simulink model "gm_parallel_lht_vnl"  (R2019b)
settings: Solver=FixedStepDiscrete  StartTime=0.0  StopTime=inf  RelTol=1e-3
undefined symbols (not defined in the file or in its folder): bt, height, nTheta, width
libraries: hdlsllib x199, simulink x27, hdlmdlgenlib x7, dspsrcs4 x1
(part 18 of 19)

== system gm_parallel_lht_vnl/Parallel LHT/Parallel LHT Kernel/Hough Kernel/Hough Kernel Symmetric Look Ahead/Look Ahead Hough/Register Bank_instance32 ==
  Data In : Inport  OutDataTypeStr=fixdt(1, 9, 0)  PortDimensions=1  SampleTime=6.66666666666667e-09
  Write Enable : Inport  Port=2  OutDataTypeStr=boolean  PortDimensions=1  SampleTime=6.66666666666667e-09
  Delay_Switch : Switch  Criteria=u2 ~= 0  Threshold=double(0)  OutDataTypeStr=fixdt(1, 9, 0)  SampleTime=6.66666666666667e-09
  Unit Delay Enabled Synchronous_lowered : Delay  DelayLength=double(1)  InitialCondition=0  SampleTime=6.66666666666667e-09
  Data Out : Outport
  wires:
  Unit Delay Enabled Synchronous_lowered/1 -> Data Out/1, Delay_Switch/3
  Data In/1 -> Delay_Switch/1
  Write Enable/1 -> Delay_Switch/2
  Delay_Switch/1 -> Unit Delay Enabled Synchronous_lowered/1

== system gm_parallel_lht_vnl/Parallel LHT/Parallel LHT Kernel/Hough Kernel/Hough Kernel Symmetric Look Ahead/Look Ahead Hough/Register Bank_instance33 ==
  Data In : Inport  OutDataTypeStr=fixdt(1, 9, 0)  PortDimensions=1  SampleTime=6.66666666666667e-09
  Write Enable : Inport  Port=2  OutDataTypeStr=boolean  PortDimensions=1  SampleTime=6.66666666666667e-09
  Delay_Switch : Switch  Criteria=u2 ~= 0  Threshold=double(0)  OutDataTypeStr=fixdt(1, 9, 0)  SampleTime=6.66666666666667e-09
  Unit Delay Enabled Synchronous_lowered : Delay  DelayLength=double(1)  InitialCondition=0  SampleTime=6.66666666666667e-09
  Data Out : Outport
  wires:
  Unit Delay Enabled Synchronous_lowered/1 -> Data Out/1, Delay_Switch/3
  Data In/1 -> Delay_Switch/1
  Write Enable/1 -> Delay_Switch/2
  Delay_Switch/1 -> Unit Delay Enabled Synchronous_lowered/1

== system gm_parallel_lht_vnl/Parallel LHT/Parallel LHT Kernel/Hough Kernel/Hough Kernel Symmetric Look Ahead/Look Ahead Hough/Register Bank_instance34 ==
  Data In : Inport  OutDataTypeStr=fixdt(1, 9, 0)  PortDimensions=1  SampleTime=6.66666666666667e-09
  Write Enable : Inport  Port=2  OutDataTypeStr=boolean  PortDimensions=1  SampleTime=6.66666666666667e-09
  Delay_Switch : Switch  Criteria=u2 ~= 0  Threshold=double(0)  OutDataTypeStr=fixdt(1, 9, 0)  SampleTime=6.66666666666667e-09
  Unit Delay Enabled Synchronous_lowered : Delay  DelayLength=double(1)  InitialCondition=0  SampleTime=6.66666666666667e-09
  Data Out : Outport
  wires:
  Unit Delay Enabled Synchronous_lowered/1 -> Data Out/1, Delay_Switch/3
  Data In/1 -> Delay_Switch/1
  Write Enable/1 -> Delay_Switch/2
  Delay_Switch/1 -> Unit Delay Enabled Synchronous_lowered/1

== system gm_parallel_lht_vnl/Parallel LHT/Parallel LHT Kernel/Hough Kernel/Hough Kernel Symmetric Look Ahead/Look Ahead Hough/Register Bank_instance35 ==
  Data In : Inport  OutDataTypeStr=fixdt(1, 9, 0)  PortDimensions=1  SampleTime=6.66666666666667e-09
  Write Enable : Inport  Port=2  OutDataTypeStr=boolean  PortDimensions=1  SampleTime=6.66666666666667e-09
  Delay_Switch : Switch  Criteria=u2 ~= 0  Threshold=double(0)  OutDataTypeStr=fixdt(1, 9, 0)  SampleTime=6.66666666666667e-09
  Unit Delay Enabled Synchronous_lowered : Delay  DelayLength=double(1)  InitialCondition=0  SampleTime=6.66666666666667e-09
  Data Out : Outport
  wires:
  Unit Delay Enabled Synchronous_lowered/1 -> Data Out/1, Delay_Switch/3
  Data In/1 -> Delay_Switch/1
  Write Enable/1 -> Delay_Switch/2
  Delay_Switch/1 -> Unit Delay Enabled Synchronous_lowered/1

== system gm_parallel_lht_vnl/Parallel LHT/Parallel LHT Kernel/Hough Kernel/Hough Kernel Symmetric Look Ahead/Look Ahead Hough/Register Bank_instance36 ==
  Data In : Inport  OutDataTypeStr=fixdt(1, 9, 0)  PortDimensions=1  SampleTime=6.66666666666667e-09
  Write Enable : Inport  Port=2  OutDataTypeStr=boolean  PortDimensions=1  SampleTime=6.66666666666667e-09
  Delay_Switch : Switch  Criteria=u2 ~= 0  Threshold=double(0)  OutDataTypeStr=fixdt(1, 9, 0)  SampleTime=6.66666666666667e-09
  Unit Delay Enabled Synchronous_lowered : Delay  DelayLength=double(1)  InitialCondition=0  SampleTime=6.66666666666667e-09
  Data Out : Outport
  wires:
  Unit Delay Enabled Synchronous_lowered/1 -> Data Out/1, Delay_Switch/3
  Data In/1 -> Delay_Switch/1
  Write Enable/1 -> Delay_Switch/2
  Delay_Switch/1 -> Unit Delay Enabled Synchronous_lowered/1

== system gm_parallel_lht_vnl/Parallel LHT/Parallel LHT Kernel/Hough Kernel/Hough Kernel Symmetric Look Ahead/Look Ahead Hough/Register Bank_instance37 ==
  Data In : Inport  OutDataTypeStr=fixdt(1, 9, 0)  PortDimensions=1  SampleTime=6.66666666666667e-09
  Write Enable : Inport  Port=2  OutDataTypeStr=boolean  PortDimensions=1  SampleTime=6.66666666666667e-09
  Delay_Switch : Switch  Criteria=u2 ~= 0  Threshold=double(0)  OutDataTypeStr=fixdt(1, 9, 0)  SampleTime=6.66666666666667e-09
  Unit Delay Enabled Synchronous_lowered : Delay  DelayLength=double(1)  InitialCondition=0  SampleTime=6.66666666666667e-09
  Data Out : Outport
  wires:
  Unit Delay Enabled Synchronous_lowered/1 -> Data Out/1, Delay_Switch/3
  Data In/1 -> Delay_Switch/1
  Write Enable/1 -> Delay_Switch/2
  Delay_Switch/1 -> Unit Delay Enabled Synchronous_lowered/1

== system gm_parallel_lht_vnl/Parallel LHT/Parallel LHT Kernel/Hough Kernel/Hough Kernel Symmetric Look Ahead/Look Ahead Hough/Register Bank_instance38 ==
  Data In : Inport  OutDataTypeStr=fixdt(1, 9, 0)  PortDimensions=1  SampleTime=6.66666666666667e-09
  Write Enable : Inport  Port=2  OutDataTypeStr=boolean  PortDimensions=1  SampleTime=6.66666666666667e-09
  Delay_Switch : Switch  Criteria=u2 ~= 0  Threshold=double(0)  OutDataTypeStr=fixdt(1, 9, 0)  SampleTime=6.66666666666667e-09
  Unit Delay Enabled Synchronous_lowered : Delay  DelayLength=double(1)  InitialCondition=0  SampleTime=6.66666666666667e-09
  Data Out : Outport
  wires:
  Unit Delay Enabled Synchronous_lowered/1 -> Data Out/1, Delay_Switch/3
  Data In/1 -> Delay_Switch/1
  Write Enable/1 -> Delay_Switch/2
  Delay_Switch/1 -> Unit Delay Enabled Synchronous_lowered/1

== system gm_parallel_lht_vnl/Parallel LHT/Parallel LHT Kernel/Hough Kernel/Hough Kernel Symmetric Look Ahead/Look Ahead Hough/Register Bank_instance39 ==
  Data In : Inport  OutDataTypeStr=fixdt(1, 9, 0)  PortDimensions=1  SampleTime=6.66666666666667e-09
  Write Enable : Inport  Port=2  OutDataTypeStr=boolean  PortDimensions=1  SampleTime=6.66666666666667e-09
  Delay_Switch : Switch  Criteria=u2 ~= 0  Threshold=double(0)  OutDataTypeStr=fixdt(1, 9, 0)  SampleTime=6.66666666666667e-09
  Unit Delay Enabled Synchronous_lowered : Delay  DelayLength=double(1)  InitialCondition=0  SampleTime=6.66666666666667e-09
  Data Out : Outport
  wires:
  Unit Delay Enabled Synchronous_lowered/1 -> Data Out/1, Delay_Switch/3
  Data In/1 -> Delay_Switch/1
  Write Enable/1 -> Delay_Switch/2
  Delay_Switch/1 -> Unit Delay Enabled Synchronous_lowered/1

== system gm_parallel_lht_vnl/Parallel LHT/Parallel LHT Kernel/Hough Kernel/Hough Kernel Symmetric Look Ahead/Look Ahead Hough/Register Bank_instance4 ==
  Data In : Inport  OutDataTypeStr=fixdt(1, 9, 0)  PortDimensions=1  SampleTime=6.66666666666667e-09
  Write Enable : Inport  Port=2  OutDataTypeStr=boolean  PortDimensions=1  SampleTime=6.66666666666667e-09
  Delay_Switch : Switch  Criteria=u2 ~= 0  Threshold=double(0)  OutDataTypeStr=fixdt(1, 9, 0)  SampleTime=6.66666666666667e-09
  Unit Delay Enabled Synchronous_lowered : Delay  DelayLength=double(1)  InitialCondition=0  SampleTime=6.66666666666667e-09
  Data Out : Outport
  wires:
  Unit Delay Enabled Synchronous_lowered/1 -> Data Out/1, Delay_Switch/3
  Data In/1 -> Delay_Switch/1
  Write Enable/1 -> Delay_Switch/2
  Delay_Switch/1 -> Unit Delay Enabled Synchronous_lowered/1

== system gm_parallel_lht_vnl/Parallel LHT/Parallel LHT Kernel/Hough Kernel/Hough Kernel Symmetric Look Ahead/Look Ahead Hough/Register Bank_instance40 ==
  Data In : Inport  OutDataTypeStr=fixdt(1, 9, 0)  PortDimensions=1  SampleTime=6.66666666666667e-09
  Write Enable : Inport  Port=2  OutDataTypeStr=boolean  PortDimensions=1  SampleTime=6.66666666666667e-09
  Delay_Switch : Switch  Criteria=u2 ~= 0  Threshold=double(0)  OutDataTypeStr=fixdt(1, 9, 0)  SampleTime=6.66666666666667e-09
  Unit Delay Enabled Synchronous_lowered : Delay  DelayLength=double(1)  InitialCondition=0  SampleTime=6.66666666666667e-09
  Data Out : Outport
  wires:
  Unit Delay Enabled Synchronous_lowered/1 -> Data Out/1, Delay_Switch/3
  Data In/1 -> Delay_Switch/1
  Write Enable/1 -> Delay_Switch/2
  Delay_Switch/1 -> Unit Delay Enabled Synchronous_lowered/1

== system gm_parallel_lht_vnl/Parallel LHT/Parallel LHT Kernel/Hough Kernel/Hough Kernel Symmetric Look Ahead/Look Ahead Hough/Register Bank_instance41 ==
  Data In : Inport  OutDataTypeStr=fixdt(1, 9, 0)  PortDimensions=1  SampleTime=6.66666666666667e-09
  Write Enable : Inport  Port=2  OutDataTypeStr=boolean  PortDimensions=1  SampleTime=6.66666666666667e-09
  Delay_Switch : Switch  Criteria=u2 ~= 0  Threshold=double(0)  OutDataTypeStr=fixdt(1, 9, 0)  SampleTime=6.66666666666667e-09
  Unit Delay Enabled Synchronous_lowered : Delay  DelayLength=double(1)  InitialCondition=0  SampleTime=6.66666666666667e-09
  Data Out : Outport
  wires:
  Unit Delay Enabled Synchronous_lowered/1 -> Data Out/1, Delay_Switch/3
  Data In/1 -> Delay_Switch/1
  Write Enable/1 -> Delay_Switch/2
  Delay_Switch/1 -> Unit Delay Enabled Synchronous_lowered/1

== system gm_parallel_lht_vnl/Parallel LHT/Parallel LHT Kernel/Hough Kernel/Hough Kernel Symmetric Look Ahead/Look Ahead Hough/Register Bank_instance42 ==
  Data In : Inport  OutDataTypeStr=fixdt(1, 9, 0)  PortDimensions=1  SampleTime=6.66666666666667e-09
  Write Enable : Inport  Port=2  OutDataTypeStr=boolean  PortDimensions=1  SampleTime=6.66666666666667e-09
  Delay_Switch : Switch  Criteria=u2 ~= 0  Threshold=double(0)  OutDataTypeStr=fixdt(1, 9, 0)  SampleTime=6.66666666666667e-09
  Unit Delay Enabled Synchronous_lowered : Delay  DelayLength=double(1)  InitialCondition=0  SampleTime=6.66666666666667e-09
  Data Out : Outport
  wires:
  Unit Delay Enabled Synchronous_lowered/1 -> Data Out/1, Delay_Switch/3
  Data In/1 -> Delay_Switch/1
  Write Enable/1 -> Delay_Switch/2
  Delay_Switch/1 -> Unit Delay Enabled Synchronous_lowered/1

== system gm_parallel_lht_vnl/Parallel LHT/Parallel LHT Kernel/Hough Kernel/Hough Kernel Symmetric Look Ahead/Look Ahead Hough/Register Bank_instance43 ==
  Data In : Inport  OutDataTypeStr=fixdt(1, 9, 0)  PortDimensions=1  SampleTime=6.66666666666667e-09
  Write Enable : Inport  Port=2  OutDataTypeStr=boolean  PortDimensions=1  SampleTime=6.66666666666667e-09
  Delay_Switch : Switch  Criteria=u2 ~= 0  Threshold=double(0)  OutDataTypeStr=fixdt(1, 9, 0)  SampleTime=6.66666666666667e-09
  Unit Delay Enabled Synchronous_lowered : Delay  DelayLength=double(1)  InitialCondition=0  SampleTime=6.66666666666667e-09
  Data Out : Outport
  wires:
  Unit Delay Enabled Synchronous_lowered/1 -> Data Out/1, Delay_Switch/3
  Data In/1 -> Delay_Switch/1
  Write Enable/1 -> Delay_Switch/2
  Delay_Switch/1 -> Unit Delay Enabled Synchronous_lowered/1

== system gm_parallel_lht_vnl/Parallel LHT/Parallel LHT Kernel/Hough Kernel/Hough Kernel Symmetric Look Ahead/Look Ahead Hough/Register Bank_instance44 ==
  Data In : Inport  OutDataTypeStr=fixdt(1, 9, 0)  PortDimensions=1  SampleTime=6.66666666666667e-09
  Write Enable : Inport  Port=2  OutDataTypeStr=boolean  PortDimensions=1  SampleTime=6.66666666666667e-09
  Delay_Switch : Switch  Criteria=u2 ~= 0  Threshold=double(0)  OutDataTypeStr=fixdt(1, 9, 0)  SampleTime=6.66666666666667e-09
  Unit Delay Enabled Synchronous_lowered : Delay  DelayLength=double(1)  InitialCondition=0  SampleTime=6.66666666666667e-09
  Data Out : Outport
  wires:
  Unit Delay Enabled Synchronous_lowered/1 -> Data Out/1, Delay_Switch/3
  Data In/1 -> Delay_Switch/1
  Write Enable/1 -> Delay_Switch/2
  Delay_Switch/1 -> Unit Delay Enabled Synchronous_lowered/1

== system gm_parallel_lht_vnl/Parallel LHT/Parallel LHT Kernel/Hough Kernel/Hough Kernel Symmetric Look Ahead/Look Ahead Hough/Register Bank_instance45 ==
  Data In : Inport  OutDataTypeStr=fixdt(1, 9, 0)  PortDimensions=1  SampleTime=6.66666666666667e-09
  Write Enable : Inport  Port=2  OutDataTypeStr=boolean  PortDimensions=1  SampleTime=6.66666666666667e-09
  Delay_Switch : Switch  Criteria=u2 ~= 0  Threshold=double(0)  OutDataTypeStr=fixdt(1, 9, 0)  SampleTime=6.66666666666667e-09
  Unit Delay Enabled Synchronous_lowered : Delay  DelayLength=double(1)  InitialCondition=0  SampleTime=6.66666666666667e-09
  Data Out : Outport
  wires:
  Unit Delay Enabled Synchronous_lowered/1 -> Data Out/1, Delay_Switch/3
  Data In/1 -> Delay_Switch/1
  Write Enable/1 -> Delay_Switch/2
  Delay_Switch/1 -> Unit Delay Enabled Synchronous_lowered/1

== system gm_parallel_lht_vnl/Parallel LHT/Parallel LHT Kernel/Hough Kernel/Hough Kernel Symmetric Look Ahead/Look Ahead Hough/Register Bank_instance46 ==
  Data In : Inport  OutDataTypeStr=fixdt(1, 9, 0)  PortDimensions=1  SampleTime=6.66666666666667e-09
  Write Enable : Inport  Port=2  OutDataTypeStr=boolean  PortDimensions=1  SampleTime=6.66666666666667e-09
  Delay_Switch : Switch  Criteria=u2 ~= 0  Threshold=double(0)  OutDataTypeStr=fixdt(1, 9, 0)  SampleTime=6.66666666666667e-09
  Unit Delay Enabled Synchronous_lowered : Delay  DelayLength=double(1)  InitialCondition=0  SampleTime=6.66666666666667e-09
  Data Out : Outport
  wires:
  Unit Delay Enabled Synchronous_lowered/1 -> Data Out/1, Delay_Switch/3
  Data In/1 -> Delay_Switch/1
  Write Enable/1 -> Delay_Switch/2
  Delay_Switch/1 -> Unit Delay Enabled Synchronous_lowered/1

== system gm_parallel_lht_vnl/Parallel LHT/Parallel LHT Kernel/Hough Kernel/Hough Kernel Symmetric Look Ahead/Look Ahead Hough/Register Bank_instance47 ==
  Data In : Inport  OutDataTypeStr=fixdt(1, 9, 0)  PortDimensions=1  SampleTime=6.66666666666667e-09
  Write Enable : Inport  Port=2  OutDataTypeStr=boolean  PortDimensions=1  SampleTime=6.66666666666667e-09
  Delay_Switch : Switch  Criteria=u2 ~= 0  Threshold=double(0)  OutDataTypeStr=fixdt(1, 9, 0)  SampleTime=6.66666666666667e-09
  Unit Delay Enabled Synchronous_lowered : Delay  DelayLength=double(1)  InitialCondition=0  SampleTime=6.66666666666667e-09
  Data Out : Outport
  wires:
  Unit Delay Enabled Synchronous_lowered/1 -> Data Out/1, Delay_Switch/3
  Data In/1 -> Delay_Switch/1
  Write Enable/1 -> Delay_Switch/2
  Delay_Switch/1 -> Unit Delay Enabled Synchronous_lowered/1

== system gm_parallel_lht_vnl/Parallel LHT/Parallel LHT Kernel/Hough Kernel/Hough Kernel Symmetric Look Ahead/Look Ahead Hough/Register Bank_instance48 ==
  Data In : Inport  OutDataTypeStr=fixdt(1, 9, 0)  PortDimensions=1  SampleTime=6.66666666666667e-09
  Write Enable : Inport  Port=2  OutDataTypeStr=boolean  PortDimensions=1  SampleTime=6.66666666666667e-09
  Delay_Switch : Switch  Criteria=u2 ~= 0  Threshold=double(0)  OutDataTypeStr=fixdt(1, 9, 0)  SampleTime=6.66666666666667e-09
  Unit Delay Enabled Synchronous_lowered : Delay  DelayLength=double(1)  InitialCondition=0  SampleTime=6.66666666666667e-09
  Data Out : Outport
  wires:
  Unit Delay Enabled Synchronous_lowered/1 -> Data Out/1, Delay_Switch/3
  Data In/1 -> Delay_Switch/1
  Write Enable/1 -> Delay_Switch/2
  Delay_Switch/1 -> Unit Delay Enabled Synchronous_lowered/1

== system gm_parallel_lht_vnl/Parallel LHT/Parallel LHT Kernel/Hough Kernel/Hough Kernel Symmetric Look Ahead/Look Ahead Hough/Register Bank_instance49 ==
  Data In : Inport  OutDataTypeStr=fixdt(1, 9, 0)  PortDimensions=1  SampleTime=6.66666666666667e-09
  Write Enable : Inport  Port=2  OutDataTypeStr=boolean  PortDimensions=1  SampleTime=6.66666666666667e-09
  Delay_Switch : Switch  Criteria=u2 ~= 0  Threshold=double(0)  OutDataTypeStr=fixdt(1, 9, 0)  SampleTime=6.66666666666667e-09
  Unit Delay Enabled Synchronous_lowered : Delay  DelayLength=double(1)  InitialCondition=0  SampleTime=6.66666666666667e-09
  Data Out : Outport
  wires:
  Unit Delay Enabled Synchronous_lowered/1 -> Data Out/1, Delay_Switch/3
  Data In/1 -> Delay_Switch/1
  Write Enable/1 -> Delay_Switch/2
  Delay_Switch/1 -> Unit Delay Enabled Synchronous_lowered/1

== system gm_parallel_lht_vnl/Parallel LHT/Parallel LHT Kernel/Hough Kernel/Hough Kernel Symmetric Look Ahead/Look Ahead Hough/Register Bank_instance5 ==
  Data In : Inport  OutDataTypeStr=fixdt(1, 9, 0)  PortDimensions=1  SampleTime=6.66666666666667e-09
  Write Enable : Inport  Port=2  OutDataTypeStr=boolean  PortDimensions=1  SampleTime=6.66666666666667e-09
  Delay_Switch : Switch  Criteria=u2 ~= 0  Threshold=double(0)  OutDataTypeStr=fixdt(1, 9, 0)  SampleTime=6.66666666666667e-09
  Unit Delay Enabled Synchronous_lowered : Delay  DelayLength=double(1)  InitialCondition=0  SampleTime=6.66666666666667e-09
  Data Out : Outport
  wires:
  Unit Delay Enabled Synchronous_lowered/1 -> Data Out/1, Delay_Switch/3
  Data In/1 -> Delay_Switch/1
  Write Enable/1 -> Delay_Switch/2
  Delay_Switch/1 -> Unit Delay Enabled Synchronous_lowered/1

== system gm_parallel_lht_vnl/Parallel LHT/Parallel LHT Kernel/Hough Kernel/Hough Kernel Symmetric Look Ahead/Look Ahead Hough/Register Bank_instance50 ==
  Data In : Inport  OutDataTypeStr=fixdt(1, 9, 0)  PortDimensions=1  SampleTime=6.66666666666667e-09
  Write Enable : Inport  Port=2  OutDataTypeStr=boolean  PortDimensions=1  SampleTime=6.66666666666667e-09
  Delay_Switch : Switch  Criteria=u2 ~= 0  Threshold=double(0)  OutDataTypeStr=fixdt(1, 9, 0)  SampleTime=6.66666666666667e-09
  Unit Delay Enabled Synchronous_lowered : Delay  DelayLength=double(1)  InitialCondition=0  SampleTime=6.66666666666667e-09
  Data Out : Outport
  wires:
  Unit Delay Enabled Synchronous_lowered/1 -> Data Out/1, Delay_Switch/3
  Data In/1 -> Delay_Switch/1
  Write Enable/1 -> Delay_Switch/2
  Delay_Switch/1 -> Unit Delay Enabled Synchronous_lowered/1

== system gm_parallel_lht_vnl/Parallel LHT/Parallel LHT Kernel/Hough Kernel/Hough Kernel Symmetric Look Ahead/Look Ahead Hough/Register Bank_instance51 ==
  Data In : Inport  OutDataTypeStr=fixdt(1, 9, 0)  PortDimensions=1  SampleTime=6.66666666666667e-09
  Write Enable : Inport  Port=2  OutDataTypeStr=boolean  PortDimensions=1  SampleTime=6.66666666666667e-09
  Delay_Switch : Switch  Criteria=u2 ~= 0  Threshold=double(0)  OutDataTypeStr=fixdt(1, 9, 0)  SampleTime=6.66666666666667e-09
  Unit Delay Enabled Synchronous_lowered : Delay  DelayLength=double(1)  InitialCondition=0  SampleTime=6.66666666666667e-09
  Data Out : Outport
  wires:
  Unit Delay Enabled Synchronous_lowered/1 -> Data Out/1, Delay_Switch/3
  Data In/1 -> Delay_Switch/1
  Write Enable/1 -> Delay_Switch/2
  Delay_Switch/1 -> Unit Delay Enabled Synchronous_lowered/1

== system gm_parallel_lht_vnl/Parallel LHT/Parallel LHT Kernel/Hough Kernel/Hough Kernel Symmetric Look Ahead/Look Ahead Hough/Register Bank_instance52 ==
  Data In : Inport  OutDataTypeStr=fixdt(1, 9, 0)  PortDimensions=1  SampleTime=6.66666666666667e-09
  Write Enable : Inport  Port=2  OutDataTypeStr=boolean  PortDimensions=1  SampleTime=6.66666666666667e-09
  Delay_Switch : Switch  Criteria=u2 ~= 0  Threshold=double(0)  OutDataTypeStr=fixdt(1, 9, 0)  SampleTime=6.66666666666667e-09
  Unit Delay Enabled Synchronous_lowered : Delay  DelayLength=double(1)  InitialCondition=0  SampleTime=6.66666666666667e-09
  Data Out : Outport
  wires:
  Unit Delay Enabled Synchronous_lowered/1 -> Data Out/1, Delay_Switch/3
  Data In/1 -> Delay_Switch/1
  Write Enable/1 -> Delay_Switch/2
  Delay_Switch/1 -> Unit Delay Enabled Synchronous_lowered/1

== system gm_parallel_lht_vnl/Parallel LHT/Parallel LHT Kernel/Hough Kernel/Hough Kernel Symmetric Look Ahead/Look Ahead Hough/Register Bank_instance53 ==
  Data In : Inport  OutDataTypeStr=fixdt(1, 9, 0)  PortDimensions=1  SampleTime=6.66666666666667e-09
  Write Enable : Inport  Port=2  OutDataTypeStr=boolean  PortDimensions=1  SampleTime=6.66666666666667e-09
  Delay_Switch : Switch  Criteria=u2 ~= 0  Threshold=double(0)  OutDataTypeStr=fixdt(1, 9, 0)  SampleTime=6.66666666666667e-09
  Unit Delay Enabled Synchronous_lowered : Delay  DelayLength=double(1)  InitialCondition=0  SampleTime=6.66666666666667e-09
  Data Out : Outport
  wires:
  Unit Delay Enabled Synchronous_lowered/1 -> Data Out/1, Delay_Switch/3
  Data In/1 -> Delay_Switch/1
  Write Enable/1 -> Delay_Switch/2
  Delay_Switch/1 -> Unit Delay Enabled Synchronous_lowered/1

== system gm_parallel_lht_vnl/Parallel LHT/Parallel LHT Kernel/Hough Kernel/Hough Kernel Symmetric Look Ahead/Look Ahead Hough/Register Bank_instance54 ==
  Data In : Inport  OutDataTypeStr=fixdt(1, 9, 0)  PortDimensions=1  SampleTime=6.66666666666667e-09
  Write Enable : Inport  Port=2  OutDataTypeStr=boolean  PortDimensions=1  SampleTime=6.66666666666667e-09
  Delay_Switch : Switch  Criteria=u2 ~= 0  Threshold=double(0)  OutDataTypeStr=fixdt(1, 9, 0)  SampleTime=6.66666666666667e-09
  Unit Delay Enabled Synchronous_lowered : Delay  DelayLength=double(1)  InitialCondition=0  SampleTime=6.66666666666667e-09
  Data Out : Outport
  wires:
  Unit Delay Enabled Synchronous_lowered/1 -> Data Out/1, Delay_Switch/3
  Data In/1 -> Delay_Switch/1
  Write Enable/1 -> Delay_Switch/2
  Delay_Switch/1 -> Unit Delay Enabled Synchronous_lowered/1

== system gm_parallel_lht_vnl/Parallel LHT/Parallel LHT Kernel/Hough Kernel/Hough Kernel Symmetric Look Ahead/Look Ahead Hough/Register Bank_instance55 ==
  Data In : Inport  OutDataTypeStr=fixdt(1, 9, 0)  PortDimensions=1  SampleTime=6.66666666666667e-09
  Write Enable : Inport  Port=2  OutDataTypeStr=boolean  PortDimensions=1  SampleTime=6.66666666666667e-09
  Delay_Switch : Switch  Criteria=u2 ~= 0  Threshold=double(0)  OutDataTypeStr=fixdt(1, 9, 0)  SampleTime=6.66666666666667e-09
  Unit Delay Enabled Synchronous_lowered : Delay  DelayLength=double(1)  InitialCondition=0  SampleTime=6.66666666666667e-09
  Data Out : Outport
  wires:
  Unit Delay Enabled Synchronous_lowered/1 -> Data Out/1, Delay_Switch/3
  Data In/1 -> Delay_Switch/1
  Write Enable/1 -> Delay_Switch/2
  Delay_Switch/1 -> Unit Delay Enabled Synchronous_lowered/1

== system gm_parallel_lht_vnl/Parallel LHT/Parallel LHT Kernel/Hough Kernel/Hough Kernel Symmetric Look Ahead/Look Ahead Hough/Register Bank_instance56 ==
  Data In : Inport  OutDataTypeStr=fixdt(1, 9, 0)  PortDimensions=1  SampleTime=6.66666666666667e-09
  Write Enable : Inport  Port=2  OutDataTypeStr=boolean  PortDimensions=1  SampleTime=6.66666666666667e-09
  Delay_Switch : Switch  Criteria=u2 ~= 0  Threshold=double(0)  OutDataTypeStr=fixdt(1, 9, 0)  SampleTime=6.66666666666667e-09
  Unit Delay Enabled Synchronous_lowered : Delay  DelayLength=double(1)  InitialCondition=0  SampleTime=6.66666666666667e-09
  Data Out : Outport
  wires:
  Unit Delay Enabled Synchronous_lowered/1 -> Data Out/1, Delay_Switch/3
  Data In/1 -> Delay_Switch/1
  Write Enable/1 -> Delay_Switch/2
  Delay_Switch/1 -> Unit Delay Enabled Synchronous_lowered/1

== system gm_parallel_lht_vnl/Parallel LHT/Parallel LHT Kernel/Hough Kernel/Hough Kernel Symmetric Look Ahead/Look Ahead Hough/Register Bank_instance57 ==
  Data In : Inport  OutDataTypeStr=fixdt(1, 9, 0)  PortDimensions=1  SampleTime=6.66666666666667e-09
  Write Enable : Inport  Port=2  OutDataTypeStr=boolean  PortDimensions=1  SampleTime=6.66666666666667e-09
  Delay_Switch : Switch  Criteria=u2 ~= 0  Threshold=double(0)  OutDataTypeStr=fixdt(1, 9, 0)  SampleTime=6.66666666666667e-09
  Unit Delay Enabled Synchronous_lowered : Delay  DelayLength=double(1)  InitialCondition=0  SampleTime=6.66666666666667e-09
  Data Out : Outport
  wires:
  Unit Delay Enabled Synchronous_lowered/1 -> Data Out/1, Delay_Switch/3
  Data In/1 -> Delay_Switch/1
  Write Enable/1 -> Delay_Switch/2
  Delay_Switch/1 -> Unit Delay Enabled Synchronous_lowered/1

== system gm_parallel_lht_vnl/Parallel LHT/Parallel LHT Kernel/Hough Kernel/Hough Kernel Symmetric Look Ahead/Look Ahead Hough/Register Bank_instance58 ==
  Data In : Inport  OutDataTypeStr=fixdt(1, 9, 0)  PortDimensions=1  SampleTime=6.66666666666667e-09
  Write Enable : Inport  Port=2  OutDataTypeStr=boolean  PortDimensions=1  SampleTime=6.66666666666667e-09
  Delay_Switch : Switch  Criteria=u2 ~= 0  Threshold=double(0)  OutDataTypeStr=fixdt(1, 9, 0)  SampleTime=6.66666666666667e-09
  Unit Delay Enabled Synchronous_lowered : Delay  DelayLength=double(1)  InitialCondition=0  SampleTime=6.66666666666667e-09
  Data Out : Outport
  wires:
  Unit Delay Enabled Synchronous_lowered/1 -> Data Out/1, Delay_Switch/3
  Data In/1 -> Delay_Switch/1
  Write Enable/1 -> Delay_Switch/2
  Delay_Switch/1 -> Unit Delay Enabled Synchronous_lowered/1

== system gm_parallel_lht_vnl/Parallel LHT/Parallel LHT Kernel/Hough Kernel/Hough Kernel Symmetric Look Ahead/Look Ahead Hough/Register Bank_instance59 ==
  Data In : Inport  OutDataTypeStr=fixdt(1, 9, 0)  PortDimensions=1  SampleTime=6.66666666666667e-09
  Write Enable : Inport  Port=2  OutDataTypeStr=boolean  PortDimensions=1  SampleTime=6.66666666666667e-09
  Delay_Switch : Switch  Criteria=u2 ~= 0  Threshold=double(0)  OutDataTypeStr=fixdt(1, 9, 0)  SampleTime=6.66666666666667e-09
  Unit Delay Enabled Synchronous_lowered : Delay  DelayLength=double(1)  InitialCondition=0  SampleTime=6.66666666666667e-09
  Data Out : Outport
  wires:
  Unit Delay Enabled Synchronous_lowered/1 -> Data Out/1, Delay_Switch/3
  Data In/1 -> Delay_Switch/1
  Write Enable/1 -> Delay_Switch/2
  Delay_Switch/1 -> Unit Delay Enabled Synchronous_lowered/1

== system gm_parallel_lht_vnl/Parallel LHT/Parallel LHT Kernel/Hough Kernel/Hough Kernel Symmetric Look Ahead/Look Ahead Hough/Register Bank_instance6 ==
  Data In : Inport  OutDataTypeStr=fixdt(1, 9, 0)  PortDimensions=1  SampleTime=6.66666666666667e-09
  Write Enable : Inport  Port=2  OutDataTypeStr=boolean  PortDimensions=1  SampleTime=6.66666666666667e-09
  Delay_Switch : Switch  Criteria=u2 ~= 0  Threshold=double(0)  OutDataTypeStr=fixdt(1, 9, 0)  SampleTime=6.66666666666667e-09
  Unit Delay Enabled Synchronous_lowered : Delay  DelayLength=double(1)  InitialCondition=0  SampleTime=6.66666666666667e-09
  Data Out : Outport
  wires:
  Unit Delay Enabled Synchronous_lowered/1 -> Data Out/1, Delay_Switch/3
  Data In/1 -> Delay_Switch/1
  Write Enable/1 -> Delay_Switch/2
  Delay_Switch/1 -> Unit Delay Enabled Synchronous_lowered/1

== system gm_parallel_lht_vnl/Parallel LHT/Parallel LHT Kernel/Hough Kernel/Hough Kernel Symmetric Look Ahead/Look Ahead Hough/Register Bank_instance60 ==
  Data In : Inport  OutDataTypeStr=fixdt(1, 9, 0)  PortDimensions=1  SampleTime=6.66666666666667e-09
  Write Enable : Inport  Port=2  OutDataTypeStr=boolean  PortDimensions=1  SampleTime=6.66666666666667e-09
  Delay_Switch : Switch  Criteria=u2 ~= 0  Threshold=double(0)  OutDataTypeStr=fixdt(1, 9, 0)  SampleTime=6.66666666666667e-09
  Unit Delay Enabled Synchronous_lowered : Delay  DelayLength=double(1)  InitialCondition=0  SampleTime=6.66666666666667e-09
  Data Out : Outport
  wires:
  Unit Delay Enabled Synchronous_lowered/1 -> Data Out/1, Delay_Switch/3
  Data In/1 -> Delay_Switch/1
  Write Enable/1 -> Delay_Switch/2
  Delay_Switch/1 -> Unit Delay Enabled Synchronous_lowered/1

== system gm_parallel_lht_vnl/Parallel LHT/Parallel LHT Kernel/Hough Kernel/Hough Kernel Symmetric Look Ahead/Look Ahead Hough/Register Bank_instance61 ==
  Data In : Inport  OutDataTypeStr=fixdt(1, 9, 0)  PortDimensions=1  SampleTime=6.66666666666667e-09
  Write Enable : Inport  Port=2  OutDataTypeStr=boolean  PortDimensions=1  SampleTime=6.66666666666667e-09
  Delay_Switch : Switch  Criteria=u2 ~= 0  Threshold=double(0)  OutDataTypeStr=fixdt(1, 9, 0)  SampleTime=6.66666666666667e-09
  Unit Delay Enabled Synchronous_lowered : Delay  DelayLength=double(1)  InitialCondition=0  SampleTime=6.66666666666667e-09
  Data Out : Outport
  wires:
  Unit Delay Enabled Synchronous_lowered/1 -> Data Out/1, Delay_Switch/3
  Data In/1 -> Delay_Switch/1
  Write Enable/1 -> Delay_Switch/2
  Delay_Switch/1 -> Unit Delay Enabled Synchronous_lowered/1

== system gm_parallel_lht_vnl/Parallel LHT/Parallel LHT Kernel/Hough Kernel/Hough Kernel Symmetric Look Ahead/Look Ahead Hough/Register Bank_instance62 ==
  Data In : Inport  OutDataTypeStr=fixdt(1, 9, 0)  PortDimensions=1  SampleTime=6.66666666666667e-09
  Write Enable : Inport  Port=2  OutDataTypeStr=boolean  PortDimensions=1  SampleTime=6.66666666666667e-09
  Delay_Switch : Switch  Criteria=u2 ~= 0  Threshold=double(0)  OutDataTypeStr=fixdt(1, 9, 0)  SampleTime=6.66666666666667e-09
  Unit Delay Enabled Synchronous_lowered : Delay  DelayLength=double(1)  InitialCondition=0  SampleTime=6.66666666666667e-09
  Data Out : Outport
  wires:
  Unit Delay Enabled Synchronous_lowered/1 -> Data Out/1, Delay_Switch/3
  Data In/1 -> Delay_Switch/1
  Write Enable/1 -> Delay_Switch/2
  Delay_Switch/1 -> Unit Delay Enabled Synchronous_lowered/1

== system gm_parallel_lht_vnl/Parallel LHT/Parallel LHT Kernel/Hough Kernel/Hough Kernel Symmetric Look Ahead/Look Ahead Hough/Register Bank_instance63 ==
  Data In : Inport  OutDataTypeStr=fixdt(1, 9, 0)  PortDimensions=1  SampleTime=6.66666666666667e-09
  Write Enable : Inport  Port=2  OutDataTypeStr=boolean  PortDimensions=1  SampleTime=6.66666666666667e-09
  Delay_Switch : Switch  Criteria=u2 ~= 0  Threshold=double(0)  OutDataTypeStr=fixdt(1, 9, 0)  SampleTime=6.66666666666667e-09
  Unit Delay Enabled Synchronous_lowered : Delay  DelayLength=double(1)  InitialCondition=0  SampleTime=6.66666666666667e-09
  Data Out : Outport
  wires:
  Unit Delay Enabled Synchronous_lowered/1 -> Data Out/1, Delay_Switch/3
  Data In/1 -> Delay_Switch/1
  Write Enable/1 -> Delay_Switch/2
  Delay_Switch/1 -> Unit Delay Enabled Synchronous_lowered/1

== system gm_parallel_lht_vnl/Parallel LHT/Parallel LHT Kernel/Hough Kernel/Hough Kernel Symmetric Look Ahead/Look Ahead Hough/Register Bank_instance64 ==
  Data In : Inport  OutDataTypeStr=fixdt(1, 9, 0)  PortDimensions=1  SampleTime=6.66666666666667e-09
  Write Enable : Inport  Port=2  OutDataTypeStr=boolean  PortDimensions=1  SampleTime=6.66666666666667e-09
  Delay_Switch : Switch  Criteria=u2 ~= 0  Threshold=double(0)  OutDataTypeStr=fixdt(1, 9, 0)  SampleTime=6.66666666666667e-09
  Unit Delay Enabled Synchronous_lowered : Delay  DelayLength=double(1)  InitialCondition=0  SampleTime=6.66666666666667e-09
  Data Out : Outport
  wires:
  Unit Delay Enabled Synchronous_lowered/1 -> Data Out/1, Delay_Switch/3
  Data In/1 -> Delay_Switch/1
  Write Enable/1 -> Delay_Switch/2
  Delay_Switch/1 -> Unit Delay Enabled Synchronous_lowered/1

== system gm_parallel_lht_vnl/Parallel LHT/Parallel LHT Kernel/Hough Kernel/Hough Kernel Symmetric Look Ahead/Look Ahead Hough/Register Bank_instance65 ==
  Data In : Inport  OutDataTypeStr=fixdt(1, 9, 0)  PortDimensions=1  SampleTime=6.66666666666667e-09
  Write Enable : Inport  Port=2  OutDataTypeStr=boolean  PortDimensions=1  SampleTime=6.66666666666667e-09
  Delay_Switch : Switch  Criteria=u2 ~= 0  Threshold=double(0)  OutDataTypeStr=fixdt(1, 9, 0)  SampleTime=6.66666666666667e-09
  Unit Delay Enabled Synchronous_lowered : Delay  DelayLength=double(1)  InitialCondition=0  SampleTime=6.66666666666667e-09
  Data Out : Outport
  wires:
  Unit Delay Enabled Synchronous_lowered/1 -> Data Out/1, Delay_Switch/3
  Data In/1 -> Delay_Switch/1
  Write Enable/1 -> Delay_Switch/2
  Delay_Switch/1 -> Unit Delay Enabled Synchronous_lowered/1

== system gm_parallel_lht_vnl/Parallel LHT/Parallel LHT Kernel/Hough Kernel/Hough Kernel Symmetric Look Ahead/Look Ahead Hough/Register Bank_instance66 ==
  Data In : Inport  OutDataTypeStr=fixdt(1, 9, 0)  PortDimensions=1  SampleTime=6.66666666666667e-09
  Write Enable : Inport  Port=2  OutDataTypeStr=boolean  PortDimensions=1  SampleTime=6.66666666666667e-09
  Delay_Switch : Switch  Criteria=u2 ~= 0  Threshold=double(0)  OutDataTypeStr=fixdt(1, 9, 0)  SampleTime=6.66666666666667e-09
  Unit Delay Enabled Synchronous_lowered : Delay  DelayLength=double(1)  InitialCondition=0  SampleTime=6.66666666666667e-09
  Data Out : Outport
  wires:
  Unit Delay Enabled Synchronous_lowered/1 -> Data Out/1, Delay_Switch/3
  Data In/1 -> Delay_Switch/1
  Write Enable/1 -> Delay_Switch/2
  Delay_Switch/1 -> Unit Delay Enabled Synchronous_lowered/1

== system gm_parallel_lht_vnl/Parallel LHT/Parallel LHT Kernel/Hough Kernel/Hough Kernel Symmetric Look Ahead/Look Ahead Hough/Register Bank_instance67 ==
  Data In : Inport  OutDataTypeStr=fixdt(1, 9, 0)  PortDimensions=1  SampleTime=6.66666666666667e-09
  Write Enable : Inport  Port=2  OutDataTypeStr=boolean  PortDimensions=1  SampleTime=6.66666666666667e-09
  Delay_Switch : Switch  Criteria=u2 ~= 0  Threshold=double(0)  OutDataTypeStr=fixdt(1, 9, 0)  SampleTime=6.66666666666667e-09
  Unit Delay Enabled Synchronous_lowered : Delay  DelayLength=double(1)  InitialCondition=0  SampleTime=6.66666666666667e-09
  Data Out : Outport
  wires:
  Unit Delay Enabled Synchronous_lowered/1 -> Data Out/1, Delay_Switch/3
  Data In/1 -> Delay_Switch/1
  Write Enable/1 -> Delay_Switch/2
  Delay_Switch/1 -> Unit Delay Enabled Synchronous_lowered/1

== system gm_parallel_lht_vnl/Parallel LHT/Parallel LHT Kernel/Hough Kernel/Hough Kernel Symmetric Look Ahead/Look Ahead Hough/Register Bank_instance68 ==
  Data In : Inport  OutDataTypeStr=fixdt(1, 9, 0)  PortDimensions=1  SampleTime=6.66666666666667e-09
  Write Enable : Inport  Port=2  OutDataTypeStr=boolean  PortDimensions=1  SampleTime=6.66666666666667e-09
  Delay_Switch : Switch  Criteria=u2 ~= 0  Threshold=double(0)  OutDataTypeStr=fixdt(1, 9, 0)  SampleTime=6.66666666666667e-09
  Unit Delay Enabled Synchronous_lowered : Delay  DelayLength=double(1)  InitialCondition=0  SampleTime=6.66666666666667e-09
  Data Out : Outport
  wires:
  Unit Delay Enabled Synchronous_lowered/1 -> Data Out/1, Delay_Switch/3
  Data In/1 -> Delay_Switch/1
  Write Enable/1 -> Delay_Switch/2
  Delay_Switch/1 -> Unit Delay Enabled Synchronous_lowered/1

== system gm_parallel_lht_vnl/Parallel LHT/Parallel LHT Kernel/Hough Kernel/Hough Kernel Symmetric Look Ahead/Look Ahead Hough/Register Bank_instance69 ==
  Data In : Inport  OutDataTypeStr=fixdt(1, 9, 0)  PortDimensions=1  SampleTime=6.66666666666667e-09
  Write Enable : Inport  Port=2  OutDataTypeStr=boolean  PortDimensions=1  SampleTime=6.66666666666667e-09
  Delay_Switch : Switch  Criteria=u2 ~= 0  Threshold=double(0)  OutDataTypeStr=fixdt(1, 9, 0)  SampleTime=6.66666666666667e-09
  Unit Delay Enabled Synchronous_lowered : Delay  DelayLength=double(1)  InitialCondition=0  SampleTime=6.66666666666667e-09
  Data Out : Outport
  wires:
  Unit Delay Enabled Synchronous_lowered/1 -> Data Out/1, Delay_Switch/3
  Data In/1 -> Delay_Switch/1
  Write Enable/1 -> Delay_Switch/2
  Delay_Switch/1 -> Unit Delay Enabled Synchronous_lowered/1

== system gm_parallel_lht_vnl/Parallel LHT/Parallel LHT Kernel/Hough Kernel/Hough Kernel Symmetric Look Ahead/Look Ahead Hough/Register Bank_instance7 ==
  Data In : Inport  OutDataTypeStr=fixdt(1, 9, 0)  PortDimensions=1  SampleTime=6.66666666666667e-09
  Write Enable : Inport  Port=2  OutDataTypeStr=boolean  PortDimensions=1  SampleTime=6.66666666666667e-09
  Delay_Switch : Switch  Criteria=u2 ~= 0  Threshold=double(0)  OutDataTypeStr=fixdt(1, 9, 0)  SampleTime=6.66666666666667e-09
  Unit Delay Enabled Synchronous_lowered : Delay  DelayLength=double(1)  InitialCondition=0  SampleTime=6.66666666666667e-09
  Data Out : Outport
  wires:
  Unit Delay Enabled Synchronous_lowered/1 -> Data Out/1, Delay_Switch/3
  Data In/1 -> Delay_Switch/1
  Write Enable/1 -> Delay_Switch/2
  Delay_Switch/1 -> Unit Delay Enabled Synchronous_lowered/1

== system gm_parallel_lht_vnl/Parallel LHT/Parallel LHT Kernel/Hough Kernel/Hough Kernel Symmetric Look Ahead/Look Ahead Hough/Register Bank_instance70 ==
  Data In : Inport  OutDataTypeStr=fixdt(1, 9, 0)  PortDimensions=1  SampleTime=6.66666666666667e-09
  Write Enable : Inport  Port=2  OutDataTypeStr=boolean  PortDimensions=1  SampleTime=6.66666666666667e-09
  Delay_Switch : Switch  Criteria=u2 ~= 0  Threshold=double(0)  OutDataTypeStr=fixdt(1, 9, 0)  SampleTime=6.66666666666667e-09
  Unit Delay Enabled Synchronous_lowered : Delay  DelayLength=double(1)  InitialCondition=0  SampleTime=6.66666666666667e-09
  Data Out : Outport
  wires:
  Unit Delay Enabled Synchronous_lowered/1 -> Data Out/1, Delay_Switch/3
  Data In/1 -> Delay_Switch/1
  Write Enable/1 -> Delay_Switch/2
  Delay_Switch/1 -> Unit Delay Enabled Synchronous_lowered/1

== system gm_parallel_lht_vnl/Parallel LHT/Parallel LHT Kernel/Hough Kernel/Hough Kernel Symmetric Look Ahead/Look Ahead Hough/Register Bank_instance71 ==
  Data In : Inport  OutDataTypeStr=fixdt(1, 9, 0)  PortDimensions=1  SampleTime=6.66666666666667e-09
  Write Enable : Inport  Port=2  OutDataTypeStr=boolean  PortDimensions=1  SampleTime=6.66666666666667e-09
  Delay_Switch : Switch  Criteria=u2 ~= 0  Threshold=double(0)  OutDataTypeStr=fixdt(1, 9, 0)  SampleTime=6.66666666666667e-09
  Unit Delay Enabled Synchronous_lowered : Delay  DelayLength=double(1)  InitialCondition=0  SampleTime=6.66666666666667e-09
  Data Out : Outport
  wires:
  Unit Delay Enabled Synchronous_lowered/1 -> Data Out/1, Delay_Switch/3
  Data In/1 -> Delay_Switch/1
  Write Enable/1 -> Delay_Switch/2
  Delay_Switch/1 -> Unit Delay Enabled Synchronous_lowered/1

== system gm_parallel_lht_vnl/Parallel LHT/Parallel LHT Kernel/Hough Kernel/Hough Kernel Symmetric Look Ahead/Look Ahead Hough/Register Bank_instance72 ==
  Data In : Inport  OutDataTypeStr=fixdt(1, 9, 0)  PortDimensions=1  SampleTime=6.66666666666667e-09
  Write Enable : Inport  Port=2  OutDataTypeStr=boolean  PortDimensions=1  SampleTime=6.66666666666667e-09
  Delay_Switch : Switch  Criteria=u2 ~= 0  Threshold=double(0)  OutDataTypeStr=fixdt(1, 9, 0)  SampleTime=6.66666666666667e-09
  Unit Delay Enabled Synchronous_lowered : Delay  DelayLength=double(1)  InitialCondition=0  SampleTime=6.66666666666667e-09
  Data Out : Outport
  wires:
  Unit Delay Enabled Synchronous_lowered/1 -> Data Out/1, Delay_Switch/3
  Data In/1 -> Delay_Switch/1
  Write Enable/1 -> Delay_Switch/2
  Delay_Switch/1 -> Unit Delay Enabled Synchronous_lowered/1

== system gm_parallel_lht_vnl/Parallel LHT/Parallel LHT Kernel/Hough Kernel/Hough Kernel Symmetric Look Ahead/Look Ahead Hough/Register Bank_instance73 ==
  Data In : Inport  OutDataTypeStr=fixdt(1, 9, 0)  PortDimensions=1  SampleTime=6.66666666666667e-09
  Write Enable : Inport  Port=2  OutDataTypeStr=boolean  PortDimensions=1  SampleTime=6.66666666666667e-09
  Delay_Switch : Switch  Criteria=u2 ~= 0  Threshold=double(0)  OutDataTypeStr=fixdt(1, 9, 0)  SampleTime=6.66666666666667e-09
  Unit Delay Enabled Synchronous_lowered : Delay  DelayLength=double(1)  InitialCondition=0  SampleTime=6.66666666666667e-09
  Data Out : Outport
  wires:
  Unit Delay Enabled Synchronous_lowered/1 -> Data Out/1, Delay_Switch/3
  Data In/1 -> Delay_Switch/1
  Write Enable/1 -> Delay_Switch/2
  Delay_Switch/1 -> Unit Delay Enabled Synchronous_lowered/1

== system gm_parallel_lht_vnl/Parallel LHT/Parallel LHT Kernel/Hough Kernel/Hough Kernel Symmetric Look Ahead/Look Ahead Hough/Register Bank_instance74 ==
  Data In : Inport  OutDataTypeStr=fixdt(1, 9, 0)  PortDimensions=1  SampleTime=6.66666666666667e-09
  Write Enable : Inport  Port=2  OutDataTypeStr=boolean  PortDimensions=1  SampleTime=6.66666666666667e-09
  Delay_Switch : Switch  Criteria=u2 ~= 0  Threshold=double(0)  OutDataTypeStr=fixdt(1, 9, 0)  SampleTime=6.66666666666667e-09
  Unit Delay Enabled Synchronous_lowered : Delay  DelayLength=double(1)  InitialCondition=0  SampleTime=6.66666666666667e-09
  Data Out : Outport
  wires:
  Unit Delay Enabled Synchronous_lowered/1 -> Data Out/1, Delay_Switch/3
  Data In/1 -> Delay_Switch/1
  Write Enable/1 -> Delay_Switch/2
  Delay_Switch/1 -> Unit Delay Enabled Synchronous_lowered/1

== system gm_parallel_lht_vnl/Parallel LHT/Parallel LHT Kernel/Hough Kernel/Hough Kernel Symmetric Look Ahead/Look Ahead Hough/Register Bank_instance75 ==
  Data In : Inport  OutDataTypeStr=fixdt(1, 9, 0)  PortDimensions=1  SampleTime=6.66666666666667e-09
  Write Enable : Inport  Port=2  OutDataTypeStr=boolean  PortDimensions=1  SampleTime=6.66666666666667e-09
  Delay_Switch : Switch  Criteria=u2 ~= 0  Threshold=double(0)  OutDataTypeStr=fixdt(1, 9, 0)  SampleTime=6.66666666666667e-09
  Unit Delay Enabled Synchronous_lowered : Delay  DelayLength=double(1)  InitialCondition=0  SampleTime=6.66666666666667e-09
  Data Out : Outport
  wires:
  Unit Delay Enabled Synchronous_lowered/1 -> Data Out/1, Delay_Switch/3
  Data In/1 -> Delay_Switch/1
  Write Enable/1 -> Delay_Switch/2
  Delay_Switch/1 -> Unit Delay Enabled Synchronous_lowered/1

== system gm_parallel_lht_vnl/Parallel LHT/Parallel LHT Kernel/Hough Kernel/Hough Kernel Symmetric Look Ahead/Look Ahead Hough/Register Bank_instance76 ==
  Data In : Inport  OutDataTypeStr=fixdt(1, 9, 0)  PortDimensions=1  SampleTime=6.66666666666667e-09
  Write Enable : Inport  Port=2  OutDataTypeStr=boolean  PortDimensions=1  SampleTime=6.66666666666667e-09
  Delay_Switch : Switch  Criteria=u2 ~= 0  Threshold=double(0)  OutDataTypeStr=fixdt(1, 9, 0)  SampleTime=6.66666666666667e-09
  Unit Delay Enabled Synchronous_lowered : Delay  DelayLength=double(1)  InitialCondition=0  SampleTime=6.66666666666667e-09
  Data Out : Outport
  wires:
  Unit Delay Enabled Synchronous_lowered/1 -> Data Out/1, Delay_Switch/3
  Data In/1 -> Delay_Switch/1
  Write Enable/1 -> Delay_Switch/2
  Delay_Switch/1 -> Unit Delay Enabled Synchronous_lowered/1

== system gm_parallel_lht_vnl/Parallel LHT/Parallel LHT Kernel/Hough Kernel/Hough Kernel Symmetric Look Ahead/Look Ahead Hough/Register Bank_instance77 ==
  Data In : Inport  OutDataTypeStr=fixdt(1, 9, 0)  PortDimensions=1  SampleTime=6.66666666666667e-09
  Write Enable : Inport  Port=2  OutDataTypeStr=boolean  PortDimensions=1  SampleTime=6.66666666666667e-09
  Delay_Switch : Switch  Criteria=u2 ~= 0  Threshold=double(0)  OutDataTypeStr=fixdt(1, 9, 0)  SampleTime=6.66666666666667e-09
  Unit Delay Enabled Synchronous_lowered : Delay  DelayLength=double(1)  InitialCondition=0  SampleTime=6.66666666666667e-09
  Data Out : Outport
  wires:
  Unit Delay Enabled Synchronous_lowered/1 -> Data Out/1, Delay_Switch/3
  Data In/1 -> Delay_Switch/1
  Write Enable/1 -> Delay_Switch/2
  Delay_Switch/1 -> Unit Delay Enabled Synchronous_lowered/1

== system gm_parallel_lht_vnl/Parallel LHT/Parallel LHT Kernel/Hough Kernel/Hough Kernel Symmetric Look Ahead/Look Ahead Hough/Register Bank_instance78 ==
  Data In : Inport  OutDataTypeStr=fixdt(1, 9, 0)  PortDimensions=1  SampleTime=6.66666666666667e-09
  Write Enable : Inport  Port=2  OutDataTypeStr=boolean  PortDimensions=1  SampleTime=6.66666666666667e-09
  Delay_Switch : Switch  Criteria=u2 ~= 0  Threshold=double(0)  OutDataTypeStr=fixdt(1, 9, 0)  SampleTime=6.66666666666667e-09
  Unit Delay Enabled Synchronous_lowered : Delay  DelayLength=double(1)  InitialCondition=0  SampleTime=6.66666666666667e-09
  Data Out : Outport
  wires:
  Unit Delay Enabled Synchronous_lowered/1 -> Data Out/1, Delay_Switch/3
  Data In/1 -> Delay_Switch/1
  Write Enable/1 -> Delay_Switch/2
  Delay_Switch/1 -> Unit Delay Enabled Synchronous_lowered/1

== system gm_parallel_lht_vnl/Parallel LHT/Parallel LHT Kernel/Hough Kernel/Hough Kernel Symmetric Look Ahead/Look Ahead Hough/Register Bank_instance79 ==
  Data In : Inport  OutDataTypeStr=fixdt(1, 9, 0)  PortDimensions=1  SampleTime=6.66666666666667e-09
  Write Enable : Inport  Port=2  OutDataTypeStr=boolean  PortDimensions=1  SampleTime=6.66666666666667e-09
  Delay_Switch : Switch  Criteria=u2 ~= 0  Threshold=double(0)  OutDataTypeStr=fixdt(1, 9, 0)  SampleTime=6.66666666666667e-09
  Unit Delay Enabled Synchronous_lowered : Delay  DelayLength=double(1)  InitialCondition=0  SampleTime=6.66666666666667e-09
  Data Out : Outport
  wires:
  Unit Delay Enabled Synchronous_lowered/1 -> Data Out/1, Delay_Switch/3
  Data In/1 -> Delay_Switch/1
  Write Enable/1 -> Delay_Switch/2
  Delay_Switch/1 -> Unit Delay Enabled Synchronous_lowered/1

== system gm_parallel_lht_vnl/Parallel LHT/Parallel LHT Kernel/Hough Kernel/Hough Kernel Symmetric Look Ahead/Look Ahead Hough/Register Bank_instance8 ==
  Data In : Inport  OutDataTypeStr=fixdt(1, 9, 0)  PortDimensions=1  SampleTime=6.66666666666667e-09
  Write Enable : Inport  Port=2  OutDataTypeStr=boolean  PortDimensions=1  SampleTime=6.66666666666667e-09
  Delay_Switch : Switch  Criteria=u2 ~= 0  Threshold=double(0)  OutDataTypeStr=fixdt(1, 9, 0)  SampleTime=6.66666666666667e-09
  Unit Delay Enabled Synchronous_lowered : Delay  DelayLength=double(1)  InitialCondition=0  SampleTime=6.66666666666667e-09
  Data Out : Outport
  wires:
  Unit Delay Enabled Synchronous_lowered/1 -> Data Out/1, Delay_Switch/3
  Data In/1 -> Delay_Switch/1
  Write Enable/1 -> Delay_Switch/2
  Delay_Switch/1 -> Unit Delay Enabled Synchronous_lowered/1

== system gm_parallel_lht_vnl/Parallel LHT/Parallel LHT Kernel/Hough Kernel/Hough Kernel Symmetric Look Ahead/Look Ahead Hough/Register Bank_instance80 ==
  Data In : Inport  OutDataTypeStr=fixdt(1, 9, 0)  PortDimensions=1  SampleTime=6.66666666666667e-09
  Write Enable : Inport  Port=2  OutDataTypeStr=boolean  PortDimensions=1  SampleTime=6.66666666666667e-09
  Delay_Switch : Switch  Criteria=u2 ~= 0  Threshold=double(0)  OutDataTypeStr=fixdt(1, 9, 0)  SampleTime=6.66666666666667e-09
  Unit Delay Enabled Synchronous_lowered : Delay  DelayLength=double(1)  InitialCondition=0  SampleTime=6.66666666666667e-09
  Data Out : Outport
  wires:
  Unit Delay Enabled Synchronous_lowered/1 -> Data Out/1, Delay_Switch/3
  Data In/1 -> Delay_Switch/1
  Write Enable/1 -> Delay_Switch/2
  Delay_Switch/1 -> Unit Delay Enabled Synchronous_lowered/1

== system gm_parallel_lht_vnl/Parallel LHT/Parallel LHT Kernel/Hough Kernel/Hough Kernel Symmetric Look Ahead/Look Ahead Hough/Register Bank_instance81 ==
  Data In : Inport  OutDataTypeStr=fixdt(1, 9, 0)  PortDimensions=1  SampleTime=6.66666666666667e-09
  Write Enable : Inport  Port=2  OutDataTypeStr=boolean  PortDimensions=1  SampleTime=6.66666666666667e-09
  Delay_Switch : Switch  Criteria=u2 ~= 0  Threshold=double(0)  OutDataTypeStr=fixdt(1, 9, 0)  SampleTime=6.66666666666667e-09
  Unit Delay Enabled Synchronous_lowered : Delay  DelayLength=double(1)  InitialCondition=0  SampleTime=6.66666666666667e-09
  Data Out : Outport
  wires:
  Unit Delay Enabled Synchronous_lowered/1 -> Data Out/1, Delay_Switch/3
  Data In/1 -> Delay_Switch/1
  Write Enable/1 -> Delay_Switch/2
  Delay_Switch/1 -> Unit Delay Enabled Synchronous_lowered/1

== system gm_parallel_lht_vnl/Parallel LHT/Parallel LHT Kernel/Hough Kernel/Hough Kernel Symmetric Look Ahead/Look Ahead Hough/Register Bank_instance82 ==
  Data In : Inport  OutDataTypeStr=fixdt(1, 9, 0)  PortDimensions=1  SampleTime=6.66666666666667e-09
  Write Enable : Inport  Port=2  OutDataTypeStr=boolean  PortDimensions=1  SampleTime=6.66666666666667e-09
  Delay_Switch : Switch  Criteria=u2 ~= 0  Threshold=double(0)  OutDataTypeStr=fixdt(1, 9, 0)  SampleTime=6.66666666666667e-09
  Unit Delay Enabled Synchronous_lowered : Delay  DelayLength=double(1)  InitialCondition=0  SampleTime=6.66666666666667e-09
  Data Out : Outport
  wires:
  Unit Delay Enabled Synchronous_lowered/1 -> Data Out/1, Delay_Switch/3
  Data In/1 -> Delay_Switch/1
  Write Enable/1 -> Delay_Switch/2
  Delay_Switch/1 -> Unit Delay Enabled Synchronous_lowered/1

== system gm_parallel_lht_vnl/Parallel LHT/Parallel LHT Kernel/Hough Kernel/Hough Kernel Symmetric Look Ahead/Look Ahead Hough/Register Bank_instance83 ==
  Data In : Inport  OutDataTypeStr=fixdt(1, 9, 0)  PortDimensions=1  SampleTime=6.66666666666667e-09
  Write Enable : Inport  Port=2  OutDataTypeStr=boolean  PortDimensions=1  SampleTime=6.66666666666667e-09
  Delay_Switch : Switch  Criteria=u2 ~= 0  Threshold=double(0)  OutDataTypeStr=fixdt(1, 9, 0)  SampleTime=6.66666666666667e-09
  Unit Delay Enabled Synchronous_lowered : Delay  DelayLength=double(1)  InitialCondition=0  SampleTime=6.66666666666667e-09
  Data Out : Outport
  wires:
  Unit Delay Enabled Synchronous_lowered/1 -> Data Out/1, Delay_Switch/3
  Data In/1 -> Delay_Switch/1
  Write Enable/1 -> Delay_Switch/2
  Delay_Switch/1 -> Unit Delay Enabled Synchronous_lowered/1

== system gm_parallel_lht_vnl/Parallel LHT/Parallel LHT Kernel/Hough Kernel/Hough Kernel Symmetric Look Ahead/Look Ahead Hough/Register Bank_instance84 ==
  Data In : Inport  OutDataTypeStr=fixdt(1, 9, 0)  PortDimensions=1  SampleTime=6.66666666666667e-09
  Write Enable : Inport  Port=2  OutDataTypeStr=boolean  PortDimensions=1  SampleTime=6.66666666666667e-09
  Delay_Switch : Switch  Criteria=u2 ~= 0  Threshold=double(0)  OutDataTypeStr=fixdt(1, 9, 0)  SampleTime=6.66666666666667e-09
  Unit Delay Enabled Synchronous_lowered : Delay  DelayLength=double(1)  InitialCondition=0  SampleTime=6.66666666666667e-09
  Data Out : Outport
  wires:
  Unit Delay Enabled Synchronous_lowered/1 -> Data Out/1, Delay_Switch/3
  Data In/1 -> Delay_Switch/1
  Write Enable/1 -> Delay_Switch/2
  Delay_Switch/1 -> Unit Delay Enabled Synchronous_lowered/1
